simulink model "cic_interp2_"  (Simulink 7.8)
settings: Solver=ode45  StartTime=0.0  StopTime=0.1  RelTol=1e-3
undefined symbols (not defined in the file or in its folder): dfilt
libraries: dspsigops x8, dspsrcs4 x1, dsparch4 x1
settings Model: Creator=svenhoffmann  LastModifiedBy=josef  ExtModeAutoUpdateStatusClock=off
settings OptimizationCC: InlineInvariantSignals=on  InitFltsAndDblsToZero=on
settings DebuggingCC: SaveWithParameterizedLinksMsg=none  SignalResolutionControl=TryResolveAllWithWarning  MultiTaskDSMMsg=warning  MultiTaskCondExecSysMsg=none  FcnCallInpInsideContextMsg=Use local settings  StrictBusMsg=None
settings RTWCC: IncludeERTFirstTime=on
settings GRTTargetCC: TargetFcnLib=ansi_tfl_tmw.mat

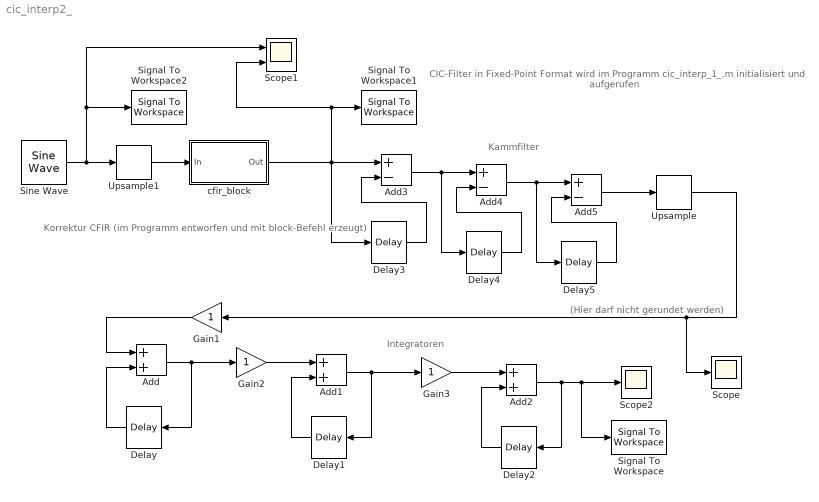
== system cic_interp2_ ==
  note: Korrektur CFIR (im Programm
      | entworfen
      | und mit block-Befehl erzeugt)
  note: CIC-Filter
      | in Fixed-Point
      | Format
      | wird im Programm cic_interp_1_.m
      | initialisiert
      | und aufgerufen
  note: Integratoren
  note: Kammfilter
  note: (Hier darf nicht gerundet werden)
  Add : Sum  OutDataTypeStr=Inherit: Same as first input
  Add1 : Sum  OutDataTypeStr=Inherit: Same as first input
  Add2 : Sum  OutDataTypeStr=Inherit: Same as first input
  Add3 : Sum  Inputs=+-
  Add4 : Sum  Inputs=+-
  Add5 : Sum  Inputs=+-
  Delay{,1..5} (6 alike) : dspsigops/Delay  InputProcessing=Inherited (this choice will be removed - see release notes)  dly_unit=Samples  delay=1  ic_detail=off  dif_ic_for_ch=off  dif_ic_for_dly=off  ic=0  reset_popup=None
  Gain1 : Gain  OutDataTypeStr=fixdt(1,19,16)
  Gain2 : Gain  OutDataTypeStr=fixdt(1,23,19)
  Gain3 : Gain  OutDataTypeStr=fixdt(1,28,24)
  Scope : Scope
  Scope1 : Scope  NumInputPorts=2
      settings: YMin=-5~-5  YMax=5~5
  Scope2 : Scope
      settings: YMin=-10  YMax=10  SaveName=ScopeData2
  Signal To Workspace : SignalToWorkspace  VariableName=yout  SaveFormat=Array
      settings: CopyFcn=dspblkcopystw(gcbh);
  Signal To Workspace1 : SignalToWorkspace  VariableName=yout1  SaveFormat=Array
      settings: CopyFcn=dspblkcopystw(gcbh);
  Signal To Workspace2 : SignalToWorkspace  VariableName=yout2  SaveFormat=Array
      settings: CopyFcn=dspblkcopystw(gcbh);  Decimation=10
  Sine Wave : dspsrcs4/Sine Wave  Amplitude=0.75  Frequency=1000/(fix(1000/50))  Phase=0  SampleMode=Discrete  OutComplex=Real  CompMethod=Table lookup  TableSize=Speed  SampleTime=1/1000  SamplesPerFrame=1  ResetState=Restart at time zero  dataType=Fixed-point  wordLen=16  udDataType=sfix(16)  fracBitsMode=User-defined  numFracBits=15  OutDataTypeStr=fixdt(1,16,15)  LastOutDataTypeStr=fixdt(1,16,15)
  Upsample : dspsigops/Upsample  N=5  phase=0  InputProcessing=Inherited (this choice will be removed - see release notes)  RateOptions=Allow multirate processing  ic=0  mode=Unused parameter value
  Upsample1 : dspsigops/Upsample  N=2  phase=0  InputProcessing=Inherited (this choice will be removed - see release notes)  RateOptions=Allow multirate processing  ic=0  mode=Unused parameter value
  cfir_block : Subsystem  Tag=BlockMethodSubSystem
  wires:
  Delay/1 -> Add/2
  Add/1 -> Delay/1, Gain2/1
  Delay1/1 -> Add1/2
  Add1/1 -> Delay1/1, Gain3/1
  Add2/1 -> Signal To Workspace/1, Scope2/1, Delay2/1
  Delay2/1 -> Add2/2
  Delay3/1 -> Add3/2
  Delay4/1 -> Add4/2
  Delay5/1 -> Add5/2
  Add3/1 -> Add4/1, Delay4/1
  Add4/1 -> Add5/1, Delay5/1
  cfir_block/1(Out) -> Add3/1, Delay3/1, Scope1/2, Signal To Workspace1/1
  Sine Wave/1 -> Upsample1/1, Signal To Workspace2/1, Scope1/1
  Add5/1 -> Upsample/1
  Upsample/1 -> Gain1/1, Scope/1
  Upsample1/1 -> cfir_block/1(In)
  Gain1/1 -> Add/1
  Gain2/1 -> Add1/1
  Gain3/1 -> Add2/1

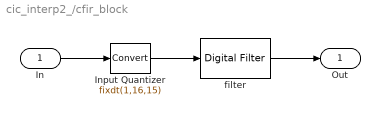
== system cic_interp2_/cfir_block ==
  In : Inport
  Input Quantizer : DataTypeConversion  OutDataTypeStr=fixdt(1,16,15)  RndMeth=Round  SaturateOnIntegerOverflow=on
  filter : dsparch4/Digital Filter  TypePopup=FIR (all zeros)  IIRFiltStruct=Direct form II transposed  AllPoleFiltStruct=Direct form  FIRFiltStruct=Direct form  CoeffSource=Specify via dialog  NumCoeffs=[0.000338712493710931 0.00118683631222087 0.00219412537230337 0.00287743030473586 0.0027642072414071 0.00142570062587514 -0.00138543448377128 -0.00554090285262467 -0.0103996092091411 -0.0147810939956912 -0.0170948285862833 -0.0156134667853961 -0.00885453127676567 0.00401692400936467 0.022857889099131 0.0463896957278871 0.072269548022093 0.0974068019367916 0.118469402697944 0.132484630872975 0.137400274946466 0.132484630872975 0.118469402697944 0.0974068019367916 0.072269548022093 0.0463896957278871 0.022857889099131 0.00401692400936467 -0.00885453127676567 -0.0156134667853961 -0.0170948285862833 -0.0147810939956912 -0.0103996092091411 -0.00554090285262467 -0.00138543448377128 0.00142570062587514 0.0027642072414071 0.00287743030473586 0.00219412537230337 0.00118683631222087 0.000338712493710931]  DenCoeffs=[1 0.1]  BiQuadCoeffs=[1 0.3 0.4 1 0.1 0.2]  LatticeCoeffs=[0.2 0.4]  denIgnore=on  FiltPerSampPopup=One filter per frame  IC=0  ICnum=0  ICden=0  firstCoeffMode=Binary point scaling  firstCoeffWordLength=16  firstCoeffFracLength=17  outputMode=Binary point scaling  outputWordLength=16  outputFracLength=15  accumMode=Binary point scaling  accumWordLength=32  accumFracLength=30  prodOutputMode=Binary point scaling  prodOutputWordLength=32  prodOutputFracLength=30  roundingMode=Floor  overflowMode=on  ScaleValues=1  scaleValueFracLength=14  stageInFracLength=15  stageOutFracLength=15  FilterSource=Specify via dialog  dfiltObjectName=dfilt.dffir([1 2 1])  InputProcessing=Columns as channels (frame based)
  Out : Outport
  wires:
  In/1 -> Input Quantizer/1
  Input Quantizer/1 -> filter/1
  filter/1 -> Out/1
